simulink model "test_vacc"  (Simulink 7.4)
settings: Solver=ode45  StartTime=0.0  StopTime=100  RelTol=1e-3
libraries: xbsIndex_r4 x40, casper_library x10, xps_library x5, isi_correlator_lib x5
settings Model: Creator=wjm  LastModifiedBy=wjm
settings OptimizationCC: InitFltsAndDblsToZero=on

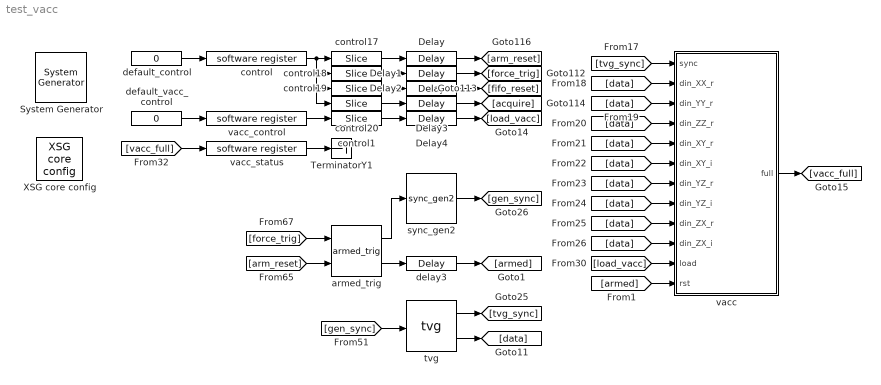
== system test_vacc ==
  " System Generator" : xbsIndex_r4/ System Generator  Tag=genX  SystemSampleTime=-1  xilinxfamily=virtex5  part=xc5vsx95t  speed=-1  package=ff1136  synthesis_tool=XST  clock_wrapper=Clock Enables  directory=./test_vacc/sysgen  testbench=off  simulink_period=1  sysclk_period=5  dcm_input_clock_period=100  incr_netlist=off  trim_vbits=Everywhere in SubSystem  dbl_ovrd=According to Block Masks  core_generation=According to Block Masks  run_coregen=off  deprecated_control=off  eval_field=0  block_type=sysgen
      settings: block_version=10.1.3
  Delay{,1..4} (5 alike) : xbsIndex_r4/Delay  en=off  latency=2  dbl_ovrd=off  reg_retiming=on  block_type=delay
      settings: block_version=11.3
  TerminatorY1 : Terminator
  XSG core config : xps_library/XSG core config  Tag=xps:xsg  SystemSampleTime=-1  hw_sys=ROACH:sx95t  ibob_linux=off  clk_src=sys_clk2x  iBOB_clk_src=sys_clk  BEE2_ctrl_clk_src=sys_clk  BEE2_usr_clk_src=sys_clk  ROACH_clk_src=sys_clk2x  CORR_clk_src=sys_clk  gpio_clk_io_group=iBOB:sma  gpio_clk_bit_index=0  clk_rate=200  sample_period=1  synthesis_tool=XST  mpc_type=powerpc440_ext
  armed_trig : isi_correlator_lib/armed_trig  SystemSampleTime=-1
  control : xps_library/software register  Tag=xps:sw_reg  SystemSampleTime=-1  io_dir=From Processor  arith_type=Unsigned  bitwidth=32  bin_pt=0  sample_period=1  gw_name=test_vacc_control_user_data_out
  control1 : xbsIndex_r4/Slice  nbits=1  boolean_output=on  mode=Lower Bit Location + Width  bit1=0  base1=MSB of Input  bit0=0  base0=LSB of Input  dbl_ovrd=off  block_type=slice
      settings: block_version=10.1.3
  control17 : xbsIndex_r4/Slice  nbits=1  boolean_output=on  mode=Lower Bit Location + Width  bit1=0  base1=MSB of Input  bit0=0  base0=LSB of Input  dbl_ovrd=off  block_type=slice
      settings: infoedit="Extracts a given range of bits from each input sample and presents it at the output.  The output type is ordinarily unsigned with binary point at zero, but can be Boolean when the slice is one bit wide.<P><P>Hardware notes: In hardware this block costs nothing."  block_version=10.1.3
  control18 : xbsIndex_r4/Slice  nbits=1  boolean_output=on  mode=Lower Bit Location + Width  bit1=0  base1=MSB of Input  bit0=1  base0=LSB of Input  dbl_ovrd=off  block_type=slice
      settings: infoedit="Extracts a given range of bits from each input sample and presents it at the output.  The output type is ordinarily unsigned with binary point at zero, but can be Boolean when the slice is one bit wide.<P><P>Hardware notes: In hardware this block costs nothing."  block_version=10.1.3
  control19 : xbsIndex_r4/Slice  nbits=1  boolean_output=on  mode=Lower Bit Location + Width  bit1=0  base1=MSB of Input  bit0=2  base0=LSB of Input  dbl_ovrd=off  block_type=slice
      settings: infoedit="Extracts a given range of bits from each input sample and presents it at the output.  The output type is ordinarily unsigned with binary point at zero, but can be Boolean when the slice is one bit wide.<P><P>Hardware notes: In hardware this block costs nothing."  block_version=10.1.3
  control20 : xbsIndex_r4/Slice  nbits=1  boolean_output=on  mode=Lower Bit Location + Width  bit1=0  base1=MSB of Input  bit0=3  base0=LSB of Input  dbl_ovrd=off  block_type=slice
      settings: infoedit="Extracts a given range of bits from each input sample and presents it at the output.  The output type is ordinarily unsigned with binary point at zero, but can be Boolean when the slice is one bit wide.<P><P>Hardware notes: In hardware this block costs nothing."  block_version=10.1.3
  default_control : Constant  Value=0  OutDataType=sfix(16)  OutScaling=2^0  SampleTime=1
  default_vacc_control : Constant  Value=0  OutDataType=sfix(16)  OutScaling=2^0  SampleTime=1
  delay3 : xbsIndex_r4/Delay  en=off  latency=1  dbl_ovrd=off  reg_retiming=off  block_type=delay
  sync_gen2 : isi_correlator_lib/sync_gen2  SystemSampleTime=-1
  tvg : isi_correlator_lib/tvg  SystemSampleTime=-1  addr_width=11
  vacc : Subsystem  AncestorBlock=isi_correlator_lib/vacc  mask{vector_length=8, out_bit_width=27, out_bin_point=4, mux_latency=2, logic_latency=2}
      mask prompts: vector_length "Vector length:"; out_bit_width "Output bit width:"; out_bin_point "Output binary point:"; mux_latency "Mux latency:"; logic_latency "Logic latency:"
  vacc_control : xps_library/software register  Tag=xps:sw_reg  SystemSampleTime=-1  io_dir=From Processor  arith_type=Unsigned  bitwidth=32  bin_pt=0  sample_period=1  gw_name=test_vacc_vacc_control_user_data_out
  vacc_status : xps_library/software register  Tag=xps:sw_reg  SystemSampleTime=-1  io_dir=To Processor  arith_type=Unsigned  bitwidth=32  bin_pt=0  sample_period=1  gw_name=test_vacc_vacc_status_user_data_in
  wires:
  control20/1 -> Delay3/1
  control19/1 -> Delay2/1
  control18/1 -> Delay1/1
  control17/1 -> Delay/1
  control/1 -> control19/1, control20/1, control18/1, control17/1
  Delay1/1 -> [force_trig]
  Delay2/1 -> [fifo_reset]
  Delay3/1 -> [acquire]
  default_control/1 -> control/1
  Delay/1 -> [arm_reset]
  armed_trig/1 -> sync_gen2/1
  [data] -> vacc/2(din_XX_r)
  [data] -> vacc/3(din_YY_r)
  [data] -> vacc/4(din_ZZ_r)
  [data] -> vacc/5(din_XY_r)
  [data] -> vacc/6(din_XY_i)
  [data] -> vacc/7(din_YZ_r)
  [data] -> vacc/8(din_YZ_i)
  [data] -> vacc/9(din_ZX_r)
  [data] -> vacc/10(din_ZX_i)
  [force_trig] -> armed_trig/1
  [arm_reset] -> armed_trig/2
  tvg/2 -> [data]
  [gen_sync] -> tvg/1
  tvg/1 -> [tvg_sync]
  sync_gen2/1 -> [gen_sync]
  [tvg_sync] -> vacc/1(sync)
  control1/1 -> Delay4/1
  Delay4/1 -> [load_vacc]
  vacc/1(full) -> [vacc_full]
  vacc_status/1 -> TerminatorY1/1
  [vacc_full] -> vacc_status/1
  default_vacc_control/1 -> vacc_control/1
  vacc_control/1 -> control1/1
  armed_trig/2 -> delay3/1
  [load_vacc] -> vacc/11(load)
  [armed] -> vacc/12(rst)
  delay3/1 -> [armed]

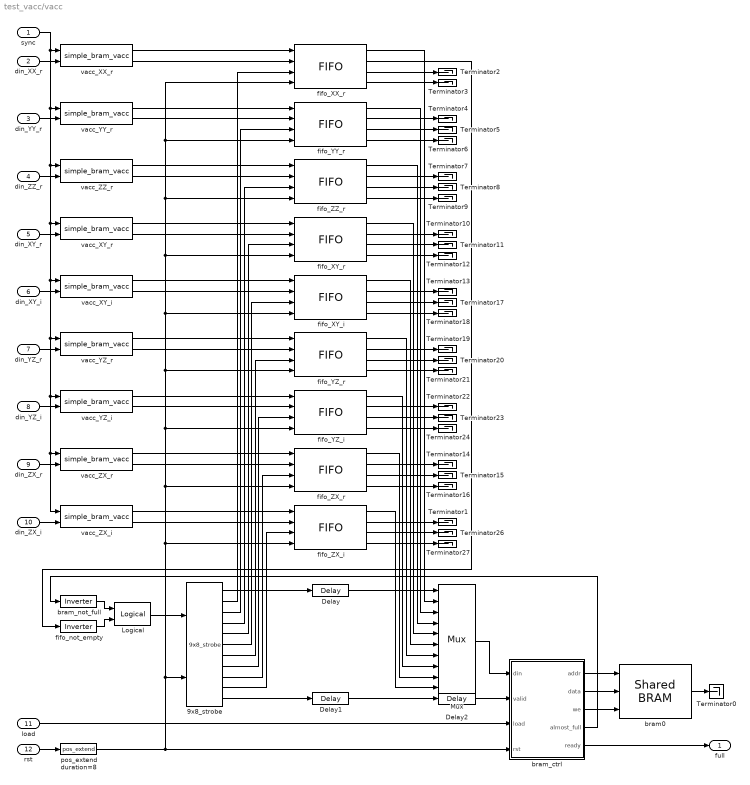
== system test_vacc/vacc ==
  sync : Inport
  din_XX_r : Inport  Port=2
  din_YY_r : Inport  Port=3
  din_ZZ_r : Inport  Port=4
  din_XY_r : Inport  Port=5
  din_XY_i : Inport  Port=6
  din_YZ_r : Inport  Port=7
  din_YZ_i : Inport  Port=8
  din_ZX_r : Inport  Port=9
  din_ZX_i : Inport  Port=10
  load : Inport  Port=11
  rst : Inport  Port=12
  9x8_strobe : isi_correlator_lib/9x8_strobe  SystemSampleTime=-1
  Delay : xbsIndex_r4/Delay  en=off  latency=1  dbl_ovrd=off  reg_retiming=off  block_type=delay
      settings: block_version=11.3
  Delay1 : xbsIndex_r4/Delay  en=off  latency=1  dbl_ovrd=off  reg_retiming=off  block_type=delay
      settings: block_version=11.3
  Delay2 : xbsIndex_r4/Delay  en=off  latency=mux_latency  dbl_ovrd=off  reg_retiming=off  block_type=delay
      settings: block_version=11.3
  Logical : xbsIndex_r4/Logical  logical_function=AND  inputs=2  en=off  latency=logic_latency  precision=Full  arith_type=Unsigned  n_bits=16  bin_pt=0  align_bp=on  dbl_ovrd=off  block_type=logical
      settings: block_version=11.3
  Mux : xbsIndex_r4/Mux  inputs=9  en=off  latency=mux_latency  precision=Full  arith_type=Unsigned  n_bits=16  bin_pt=14  quantization=Truncate  overflow=Wrap  dbl_ovrd=off  block_type=mux
      settings: block_version=11.3
  Terminator{0..24,26..27} (27 alike) : Terminator
  bram0 : xps_library/Shared BRAM  Tag=xps:bram  SystemSampleTime=-1  arith_type="Signed  (2's comp)"  addr_width=11  data_width=32  data_bin_pt=0  init_vals=0  sample_rate=1
  bram_ctrl : Subsystem  mask{output_latency=1, feedback_latency=logic_latency + 1 + mux_latency}
      mask prompts: output_latency "Output latency:"; feedback_latency "Feedback latency:"
  bram_not_full : xbsIndex_r4/Inverter  en=off  latency=0  dbl_ovrd=off  block_type=inv
      settings: block_version=11.3
  fifo_XX_r : xbsIndex_r4/FIFO  depth=512  percent_nbits=1  rst=on  en=off  use_dcount=off  use_almost_empty=off  almost_empty_thresh=2  use_almost_full=off  almost_full_thresh=14  dbl_ovrd=off  mem_type=Block RAM  explicit_period=off  block_type=fifo
      settings: block_version=11.3
  fifo_XY_i : xbsIndex_r4/FIFO  depth=512  percent_nbits=1  rst=on  en=off  use_dcount=off  use_almost_empty=off  almost_empty_thresh=2  use_almost_full=off  almost_full_thresh=14  dbl_ovrd=off  mem_type=Block RAM  explicit_period=off  block_type=fifo
      settings: block_version=11.3
  fifo_XY_r : xbsIndex_r4/FIFO  depth=512  percent_nbits=1  rst=on  en=off  use_dcount=off  use_almost_empty=off  almost_empty_thresh=2  use_almost_full=off  almost_full_thresh=14  dbl_ovrd=off  mem_type=Block RAM  explicit_period=off  block_type=fifo
      settings: block_version=11.3
  fifo_YY_r : xbsIndex_r4/FIFO  depth=512  percent_nbits=1  rst=on  en=off  use_dcount=off  use_almost_empty=off  almost_empty_thresh=2  use_almost_full=off  almost_full_thresh=14  dbl_ovrd=off  mem_type=Block RAM  explicit_period=off  block_type=fifo
      settings: block_version=11.3
  fifo_YZ_i : xbsIndex_r4/FIFO  depth=512  percent_nbits=1  rst=on  en=off  use_dcount=off  use_almost_empty=off  almost_empty_thresh=2  use_almost_full=off  almost_full_thresh=14  dbl_ovrd=off  mem_type=Block RAM  explicit_period=off  block_type=fifo
      settings: block_version=11.3
  fifo_YZ_r : xbsIndex_r4/FIFO  depth=512  percent_nbits=1  rst=on  en=off  use_dcount=off  use_almost_empty=off  almost_empty_thresh=2  use_almost_full=off  almost_full_thresh=14  dbl_ovrd=off  mem_type=Block RAM  explicit_period=off  block_type=fifo
      settings: block_version=11.3
  fifo_ZX_i : xbsIndex_r4/FIFO  depth=512  percent_nbits=1  rst=on  en=off  use_dcount=off  use_almost_empty=off  almost_empty_thresh=2  use_almost_full=off  almost_full_thresh=14  dbl_ovrd=off  mem_type=Block RAM  explicit_period=off  block_type=fifo
      settings: block_version=11.3
  fifo_ZX_r : xbsIndex_r4/FIFO  depth=512  percent_nbits=1  rst=on  en=off  use_dcount=off  use_almost_empty=off  almost_empty_thresh=2  use_almost_full=off  almost_full_thresh=14  dbl_ovrd=off  mem_type=Block RAM  explicit_period=off  block_type=fifo
      settings: block_version=11.3
  fifo_ZZ_r : xbsIndex_r4/FIFO  depth=512  percent_nbits=1  rst=on  en=off  use_dcount=off  use_almost_empty=off  almost_empty_thresh=2  use_almost_full=off  almost_full_thresh=14  dbl_ovrd=off  mem_type=Block RAM  explicit_period=off  block_type=fifo
      settings: block_version=11.3
  fifo_not_empty : xbsIndex_r4/Inverter  en=off  latency=0  dbl_ovrd=off  block_type=inv
      settings: block_version=11.3
  pos_extend duration=8 : isi_correlator_lib/pos_extend  SystemSampleTime=-1  duration=8
  vacc_XX_r : casper_library/Accumulators/simple_bram_vacc  SystemSampleTime=-1  n_chans=vector_length  n_bits=out_bit_width  bin_pos=out_bin_point
  vacc_XY_i : casper_library/Accumulators/simple_bram_vacc  SystemSampleTime=-1  n_chans=vector_length  n_bits=out_bit_width  bin_pos=out_bin_point
  vacc_XY_r : casper_library/Accumulators/simple_bram_vacc  SystemSampleTime=-1  n_chans=vector_length  n_bits=out_bit_width  bin_pos=out_bin_point
  vacc_YY_r : casper_library/Accumulators/simple_bram_vacc  SystemSampleTime=-1  n_chans=vector_length  n_bits=out_bit_width  bin_pos=out_bin_point
  vacc_YZ_i : casper_library/Accumulators/simple_bram_vacc  SystemSampleTime=-1  n_chans=vector_length  n_bits=out_bit_width  bin_pos=out_bin_point
  vacc_YZ_r : casper_library/Accumulators/simple_bram_vacc  SystemSampleTime=-1  n_chans=vector_length  n_bits=out_bit_width  bin_pos=out_bin_point
  vacc_ZX_i : casper_library/Accumulators/simple_bram_vacc  SystemSampleTime=-1  n_chans=vector_length  n_bits=out_bit_width  bin_pos=out_bin_point
  vacc_ZX_r : casper_library/Accumulators/simple_bram_vacc  SystemSampleTime=-1  n_chans=vector_length  n_bits=out_bit_width  bin_pos=out_bin_point
  vacc_ZZ_r : casper_library/Accumulators/simple_bram_vacc  SystemSampleTime=-1  n_chans=vector_length  n_bits=out_bit_width  bin_pos=out_bin_point
  full : Outport
  wires:
  fifo_not_empty/1 -> Logical/2
  bram_not_full/1 -> Logical/1
  Logical/1 -> 9x8_strobe/1
  rst/1 -> pos_extend duration=8/1
  Mux/1 -> bram_ctrl/1(din)
  fifo_XX_r/2 -> fifo_not_empty/1
  bram_ctrl/3(we) -> bram0/3
  bram_ctrl/2(data) -> bram0/2
  bram_ctrl/1(addr) -> bram0/1
  Delay2/1 -> bram_ctrl/2(valid)
  bram0/1 -> Terminator0/1
  fifo_ZX_i/1 -> Mux/10
  fifo_ZX_r/1 -> Mux/9
  fifo_YZ_i/1 -> Mux/8
  fifo_YZ_r/1 -> Mux/7
  fifo_XY_i/1 -> Mux/6
  fifo_XY_r/1 -> Mux/5
  fifo_ZZ_r/1 -> Mux/4
  fifo_YY_r/1 -> Mux/3
  fifo_XX_r/1 -> Mux/2
  9x8_strobe/10 -> fifo_ZX_i/3
  9x8_strobe/9 -> fifo_ZX_r/3
  9x8_strobe/8 -> fifo_YZ_i/3
  9x8_strobe/7 -> fifo_YZ_r/3
  9x8_strobe/6 -> fifo_XY_i/3
  9x8_strobe/5 -> fifo_XY_r/3
  9x8_strobe/4 -> fifo_ZZ_r/3
  9x8_strobe/3 -> fifo_YY_r/3
  fifo_ZX_i/4 -> Terminator27/1
  fifo_ZX_i/3 -> Terminator26/1
  fifo_ZX_r/4 -> Terminator16/1
  fifo_ZX_r/3 -> Terminator15/1
  fifo_ZX_r/2 -> Terminator14/1
  fifo_YZ_i/4 -> Terminator24/1
  fifo_YZ_i/3 -> Terminator23/1
  fifo_YZ_i/2 -> Terminator22/1
  fifo_YZ_r/4 -> Terminator21/1
  fifo_YZ_r/3 -> Terminator20/1
  fifo_YZ_r/2 -> Terminator19/1
  fifo_XY_i/4 -> Terminator18/1
  fifo_XY_i/3 -> Terminator17/1
  fifo_XY_i/2 -> Terminator13/1
  fifo_XY_r/4 -> Terminator12/1
  fifo_XY_r/3 -> Terminator11/1
  fifo_XY_r/2 -> Terminator10/1
  fifo_ZZ_r/4 -> Terminator9/1
  fifo_ZZ_r/3 -> Terminator8/1
  fifo_ZZ_r/2 -> Terminator7/1
  fifo_YY_r/4 -> Terminator6/1
  fifo_YY_r/3 -> Terminator5/1
  fifo_YY_r/2 -> Terminator4/1
  fifo_XX_r/4 -> Terminator3/1
  fifo_XX_r/3 -> Terminator2/1
  Delay1/1 -> Delay2/1
  Delay/1 -> Mux/1
  9x8_strobe/11 -> Delay1/1
  9x8_strobe/1 -> Delay/1
  vacc_ZX_i/2 -> fifo_ZX_i/2
  vacc_ZX_i/1 -> fifo_ZX_i/1
  vacc_ZX_r/2 -> fifo_ZX_r/2
  vacc_ZX_r/1 -> fifo_ZX_r/1
  vacc_YZ_i/2 -> fifo_YZ_i/2
  vacc_YZ_i/1 -> fifo_YZ_i/1
  vacc_YZ_r/2 -> fifo_YZ_r/2
  vacc_YZ_r/1 -> fifo_YZ_r/1
  vacc_XY_i/2 -> fifo_XY_i/2
  vacc_XY_i/1 -> fifo_XY_i/1
  vacc_XY_r/2 -> fifo_XY_r/2
  vacc_XY_r/1 -> fifo_XY_r/1
  vacc_ZZ_r/2 -> fifo_ZZ_r/2
  vacc_ZZ_r/1 -> fifo_ZZ_r/1
  vacc_YY_r/2 -> fifo_YY_r/2
  vacc_YY_r/1 -> fifo_YY_r/1
  vacc_XX_r/2 -> fifo_XX_r/2
  vacc_XX_r/1 -> fifo_XX_r/1
  din_ZX_i/1 -> vacc_ZX_i/2
  din_ZX_r/1 -> vacc_ZX_r/2
  din_YZ_i/1 -> vacc_YZ_i/2
  din_YZ_r/1 -> vacc_YZ_r/2
  din_XY_i/1 -> vacc_XY_i/2
  din_XY_r/1 -> vacc_XY_r/2
  din_ZZ_r/1 -> vacc_ZZ_r/2
  din_YY_r/1 -> vacc_YY_r/2
  din_XX_r/1 -> vacc_XX_r/2
  sync/1 -> vacc_XX_r/1, vacc_YY_r/1, vacc_ZZ_r/1, vacc_XY_r/1, vacc_XY_i/1, vacc_YZ_r/1, vacc_YZ_i/1, vacc_ZX_r/1, vacc_ZX_i/1
  fifo_ZX_i/2 -> Terminator1/1
  bram_ctrl/5(ready) -> full/1
  9x8_strobe/2 -> fifo_XX_r/3
  bram_ctrl/4(almost_full) -> bram_not_full/1
  pos_extend duration=8/1 -> fifo_XX_r/4, fifo_YY_r/4, fifo_ZZ_r/4, fifo_XY_r/4, fifo_XY_i/4, fifo_YZ_r/4, fifo_YZ_i/4, fifo_ZX_r/4, fifo_ZX_i/4, 9x8_strobe/2, bram_ctrl/4(rst)
  load/1 -> bram_ctrl/3(load)

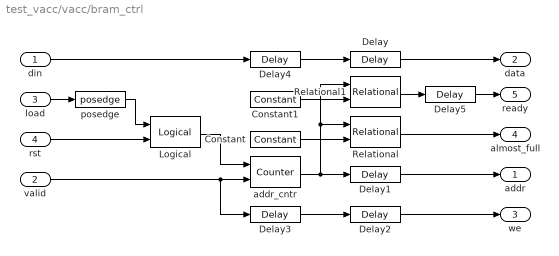
== system test_vacc/vacc/bram_ctrl ==
  din : Inport
  valid : Inport  Port=2
  load : Inport  Port=3
  rst : Inport  Port=4
  Constant : xbsIndex_r4/Constant  arith_type=Unsigned  const=72*floor(2^11/72) - 1 - (output_latency + feedback_latency)  n_bits=11  bin_pt=0  explicit_period=on  period=1  equ=P=C  opselect=C  inp2=PCIN>>17  opr=+  inp1=P  carry=CIN  dbl_ovrd=off  block_type=constant
      settings: block_version=11.3
  Constant1 : xbsIndex_r4/Constant  arith_type=Unsigned  const=72*floor(2^11/72) - 1  n_bits=11  bin_pt=0  explicit_period=on  period=1  equ=P=C  opselect=C  inp2=PCIN>>17  opr=+  inp1=P  carry=CIN  dbl_ovrd=off  block_type=constant
      settings: block_version=11.3
  Delay : xbsIndex_r4/Delay  en=off  latency=output_latency  dbl_ovrd=off  reg_retiming=off  block_type=delay
      settings: block_version=11.3
  Delay1 : xbsIndex_r4/Delay  en=off  latency=output_latency  dbl_ovrd=off  reg_retiming=off  block_type=delay
      settings: block_version=11.3
  Delay2 : xbsIndex_r4/Delay  en=off  latency=output_latency  dbl_ovrd=off  reg_retiming=off  block_type=delay
      settings: block_version=11.3
  Delay3 : xbsIndex_r4/Delay  en=off  latency=1  dbl_ovrd=off  reg_retiming=off  block_type=delay
      settings: block_version=11.3
  Delay4 : xbsIndex_r4/Delay  en=off  latency=1  dbl_ovrd=off  reg_retiming=off  block_type=delay
      settings: block_version=11.3
  Delay5 : xbsIndex_r4/Delay  en=off  latency=1  dbl_ovrd=off  reg_retiming=off  block_type=delay
      settings: block_version=11.3
  Logical : xbsIndex_r4/Logical  logical_function=OR  inputs=2  en=off  latency=0  precision=Full  arith_type=Unsigned  n_bits=16  bin_pt=0  align_bp=on  dbl_ovrd=off  block_type=logical
      settings: block_version=11.3
  Relational : xbsIndex_r4/Relational  mode=a>=b  en=off  latency=output_latency  dbl_ovrd=off  block_type=relational
      settings: block_version=11.3
  Relational1 : xbsIndex_r4/Relational  mode=a=b  en=off  latency=output_latency  dbl_ovrd=off  block_type=relational
      settings: block_version=11.3
  addr_cntr : xbsIndex_r4/Counter  cnt_type=Free Running  cnt_to=Inf  operation=Up  start_count=0  cnt_by_val=1  arith_type=Unsigned  n_bits=11  bin_pt=0  load_pin=off  rst=on  en=on  explicit_period=on  period=1  dbl_ovrd=off  use_behavioral_HDL=off  implementation=Fabric  block_type=counter
      settings: block_version=11.3
  posedge : casper_library/Misc/posedge  Tag=Rising Edge Detector  SystemSampleTime=-1
  addr : Outport
  data : Outport  Port=2
  we : Outport  Port=3
  almost_full : Outport  Port=4
  ready : Outport  Port=5
  wires:
  Delay2/1 -> we/1
  Delay1/1 -> addr/1
  Delay/1 -> data/1
  Relational/1 -> almost_full/1
  din/1 -> Delay4/1
  addr_cntr/1 -> Delay1/1, Relational1/1, Relational/1
  valid/1 -> addr_cntr/2, Delay3/1
  Delay3/1 -> Delay2/1
  Delay4/1 -> Delay/1
  Relational1/1 -> Delay5/1
  Constant/1 -> Relational/2
  Constant1/1 -> Relational1/2
  Delay5/1 -> ready/1
  load/1 -> posedge/1
  posedge/1 -> Logical/1
  Logical/1 -> addr_cntr/1
  rst/1 -> Logical/2
